simulink model "simulacion_con_f"  (R2021a)
settings: Solver=VariableStepAuto  StartTime=0.0  StopTime=10  RelTol=1e-3
settings Model: Creator=franc  LastModifiedBy=facun

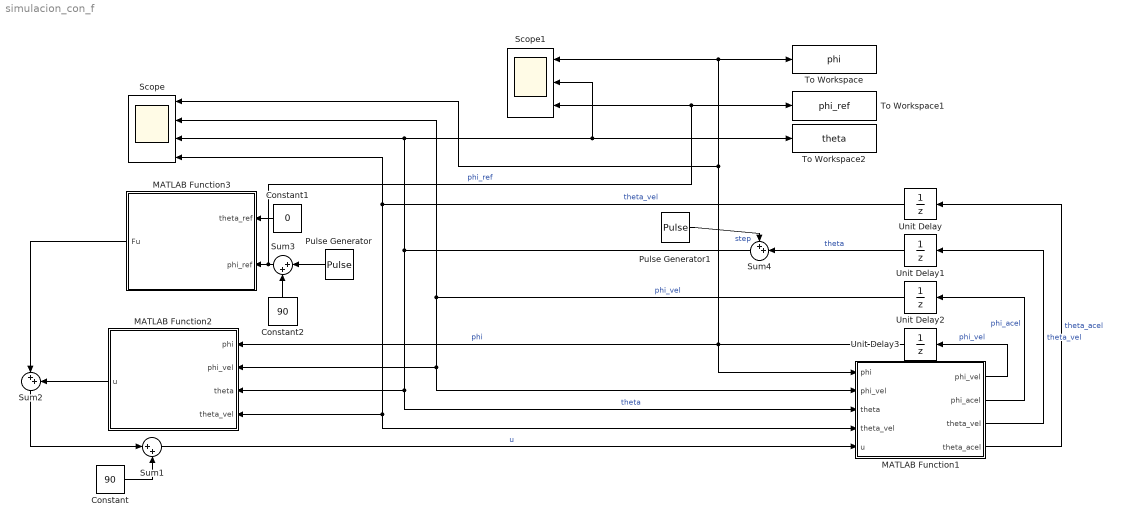
== system simulacion_con_f ==
  Constant : Constant  Value=90
  Constant1 : Constant  Value=0
  Constant2 : Constant  Value=90
  MATLAB Function1 : MATLAB Function  TreatAsAtomicUnit=on
  MATLAB Function2 : MATLAB Function  TreatAsAtomicUnit=on
  MATLAB Function3 : MATLAB Function  TreatAsAtomicUnit=on
  Pulse Generator : DiscretePulseGenerator  PulseType=Time based  Amplitude=0  Period=5  PulseWidth=50  PhaseDelay=2
  Pulse Generator1 : DiscretePulseGenerator  PulseType=Time based  Amplitude=-8  Period=5  PulseWidth=3  PhaseDelay=2
  Scope : Scope  NumInputPorts=4
  Scope1 : Scope  NumInputPorts=3
  Sum1 : Sum  Inputs=|++
  Sum2 : Sum  Inputs=|++
  Sum3 : Sum  Inputs=|++
  Sum4 : Sum  Inputs=++|
  To Workspace : ToWorkspace  VariableName=phi  SaveFormat=Timeseries  SampleTime=-1
  To Workspace1 : ToWorkspace  VariableName=phi_ref  SaveFormat=Timeseries  SampleTime=-1
  To Workspace2 : ToWorkspace  VariableName=theta  SaveFormat=Timeseries  SampleTime=-1
  Unit Delay : UnitDelay  SampleTime=0.01  HasFrameUpgradeWarning=on
  Unit Delay1 : UnitDelay  SampleTime=0.01  HasFrameUpgradeWarning=on
  Unit Delay2 : UnitDelay  SampleTime=0.01  HasFrameUpgradeWarning=on
  Unit Delay3 : UnitDelay  InitialCondition=90  SampleTime=0.01  HasFrameUpgradeWarning=on
  wires:
  MATLAB Function1/1(phi_vel) -> Unit Delay3/1  "phi_vel"
  MATLAB Function1/2(phi_acel) -> Unit Delay2/1  "phi_acel"
  Unit Delay2/1 -> MATLAB Function2/2(phi_vel), MATLAB Function1/2("phi_vel "), Scope/2  "phi_vel"
  MATLAB Function1/3(theta_vel) -> Unit Delay1/1  "theta_vel"
  MATLAB Function1/4(theta_acel) -> Unit Delay/1  "theta_acel"
  Unit Delay3/1 -> MATLAB Function2/1(phi), Scope/1, Scope1/1, To Workspace/1, MATLAB Function1/1(phi)  "phi"
  Sum1/1 -> MATLAB Function1/5(u)  "u"
  Constant/1 -> Sum1/2
  Unit Delay/1 -> MATLAB Function2/4(theta_vel), MATLAB Function1/4("theta_vel "), Scope/4  "theta_vel"
  MATLAB Function3/1(Fu) -> Sum2/1
  MATLAB Function2/1(u) -> Sum2/2
  Sum2/1 -> Sum1/1
  Constant1/1 -> MATLAB Function3/1(theta_ref)
  Sum3/1 -> To Workspace1/1, Scope1/3, MATLAB Function3/2(phi_ref)  "phi_ref"
  Pulse Generator/1 -> Sum3/1
  Constant2/1 -> Sum3/2
  Pulse Generator1/1 -> Sum4/1  "step"
  Sum4/1 -> Scope/3, To Workspace2/1, Scope1/2, MATLAB Function1/3(theta), MATLAB Function2/3(theta)  "theta"
  Unit Delay1/1 -> Sum4/2  "theta"

== matlab function simulacion_con_f/MATLAB Function1 ==
  data: phi input; phi_vel input; theta input; theta_vel input; u input; phi_vel output; phi_acel output; theta_vel output; theta_acel output
function [phi_vel,phi_acel,theta_vel,theta_acel] = fcn(phi,phi_vel,theta,theta_vel,u)

Ad = [
    1.0000    0.0100         0         0;
   -0.5765    0.9895   -2.1322   -0.2132;
         0         0    1.0000    0.0100;
         0         0   -2.5000    0.7500;
];
   
Bd = [
         0;
  2.132250;
         0;
  2.500000
];

x  = [theta theta_vel phi phi_vel];
x_dot = Ad * x' + Bd * u;
theta_vel = x_dot(1);
theta_acel = x_dot(2);
phi_vel = x_dot(3);
phi_acel = x_dot(4);

== matlab function simulacion_con_f/MATLAB Function2 ==
  data: phi input; phi_vel input; theta input; theta_vel input; u output
function u = fcn(phi,phi_vel,theta,theta_vel)
    K = [-0.5, 0.001, 0.7, -0.005];
    u = K(1) * theta + K(2) * theta_vel + K(3) * (phi - 90) + K(4) * phi_vel;

== matlab function simulacion_con_f/MATLAB Function3 ==
  data: theta_ref input; phi_ref input; Fu output
function Fu = fcn(theta_ref, phi_ref)
    F = [0, 0.3];
    Fu = F(1) * theta_ref + F(2) * (phi_ref - 90);
